simulink model "RCAM"  (R2018a)
settings: Solver=VariableStepAuto  StartTime=0.0  StopTime=60  RelTol=1e-3
undefined symbols (not defined in the file or in its folder): IC, RCAM_model
settings Model: Creator=micozmei  LastModifiedBy=micozmei

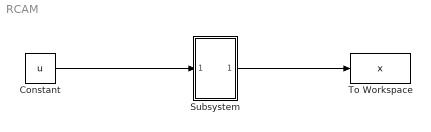
== system RCAM ==
  Constant : Constant  Value=u
  Subsystem : Subsystem
  To Workspace : ToWorkspace  VariableName=x  SaveFormat=Structure With Time  SampleTime=-1
  wires:
  Constant/1 -> Subsystem/1(In1)
  Subsystem/1(Out1) -> To Workspace/1

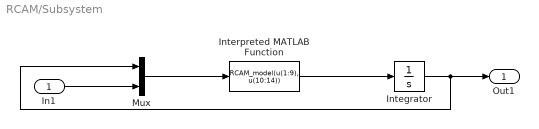
== system RCAM/Subsystem ==
  In1 : Inport
  Integrator : Integrator  InitialCondition=IC
  Interpreted MATLAB Function : MATLABFcn  MATLABFcn=RCAM_model(u(1:9), u(10:14))
  Mux : Mux  Inputs=2
  Out1 : Outport
  wires:
  Interpreted MATLAB Function/1 -> Integrator/1
  Integrator/1 -> Mux/1, Out1/1
  Mux/1 -> Interpreted MATLAB Function/1
  In1/1 -> Mux/2
